simulink model "NL_MSD_RefTrajTrac_Opti_SMC_v01"  (R2024b)
settings: Solver=VariableStepAuto  StartTime=0.0  StopTime=max(t)  RelTol=1e-3
values from neighbouring files (symbols this model uses):
  c = zeta * ccr    [Trajectory_Profile_v01.m]
  k = 1e3    (= 1000)    [Trajectory_Profile_v01.m]
  m = 1    [Trajectory_Profile_v01.m]
undefined symbols (not defined in the file or in its folder): eta, lambda
settings Model: Creator=ababaei  LastModifiedBy=ababaei

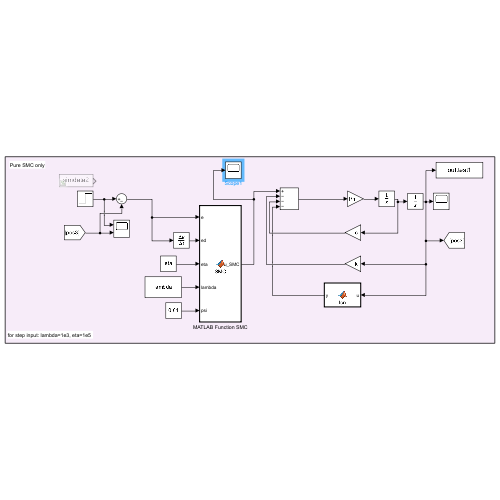
[thumbnail: Simulink's stored preview of the top-level diagram]
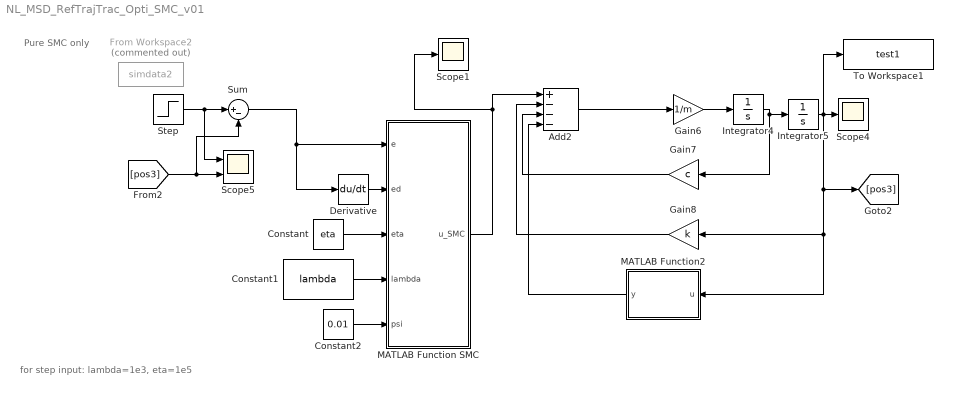
== system NL_MSD_RefTrajTrac_Opti_SMC_v01 ==
  note: for step input: lambda=1e3, eta=1e5
  note: Pure SMC only
  Add2 : Sum  Inputs=+---
  Constant : Constant  Value=eta
  Constant1 : Constant  Value=lambda
  Constant2 : Constant  Value=0.01
  Derivative : Derivative
  From Workspace2 : FromWorkspace  Commented=on  VariableName=simdata2
  Gain6 : Gain  Gain=1/m
  Gain7 : Gain  Gain=c
  Gain8 : Gain  Gain=k
  Integrator4 : Integrator
  Integrator5 : Integrator
  MATLAB Function SMC : MATLAB Function  TreatAsAtomicUnit=on
  MATLAB Function2 : MATLAB Function  TreatAsAtomicUnit=on
  Scope1 : Scope
  Scope4 : Scope
  Scope5 : Scope  NumInputPorts=2
  Step : Step  Time=0.2  SampleTime=0
  Sum : Sum  Inputs=|+-
  To Workspace1 : ToWorkspace  VariableName=test1  SaveFormat=Timeseries  SampleTime=-1
  wires:
  Gain8/1 -> Add2/2
  [pos3] -> Sum/2, Scope5/2
  Integrator5/1 -> To Workspace1/1, [pos3], MATLAB Function2/1(u), Gain8/1, Scope4/1
  Gain6/1 -> Integrator4/1
  Add2/1 -> Gain6/1
  MATLAB Function2/1(y) -> Add2/4
  Integrator4/1 -> Integrator5/1, Gain7/1
  Gain7/1 -> Add2/3
  MATLAB Function SMC/1(u_SMC) -> Scope1/1, Add2/1
  Sum/1 -> MATLAB Function SMC/1(e), Derivative/1
  Derivative/1 -> MATLAB Function SMC/2(ed)
  Constant/1 -> MATLAB Function SMC/3(eta)
  Constant1/1 -> MATLAB Function SMC/4(lambda)
  Constant2/1 -> MATLAB Function SMC/5(psi)
  Step/1 -> Scope5/1, Sum/1

== matlab function NL_MSD_RefTrajTrac_Opti_SMC_v01/MATLAB Function SMC ==
  data: e input; u_SMC output; ed input; eta input; lambda input; psi input
function u_SMC = SMC(e, ed, eta, lambda, psi)

S = ed + lambda*e; 

if abs(S) > psi
    sat_S = sign(S);
else 
    sat_S = S/psi;
end

u_SMC = -(ed - eta*sat_S);

== matlab function NL_MSD_RefTrajTrac_Opti_SMC_v01/MATLAB Function2 ==
  data: u input; y output
function y = fcn(u)
kNL = 100;
y = kNL*u;
